simulink model "longitudinal_fuzzy_LiuChang"  (R2021b)
settings: Solver=VariableStepAuto  StartTime=0.0  StopTime=60  RelTol=1e-3
libraries: commrandsrc3 x3, fuzblock x3
settings Model: Creator=dell  LastModifiedBy=lenovo
settings SolverCC: ZeroCrossAlgorithm=Adaptive  AlgebraicLoopSolver=TrustRegion
settings DebuggingCC: IgnoredZcDiagnostic=none  SFMachineParentedDataDiag=warning  ArithmeticOperatorsInVariantConditions=warning
settings SFSimCC: CustomCodeUndefinedFunction=UseInterfaceOnly

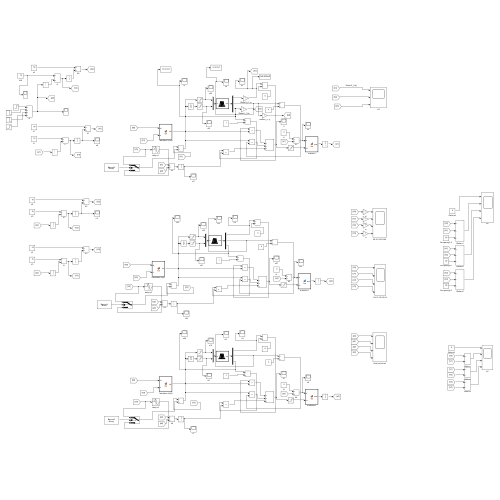
[thumbnail: Simulink's stored preview of the top-level diagram]
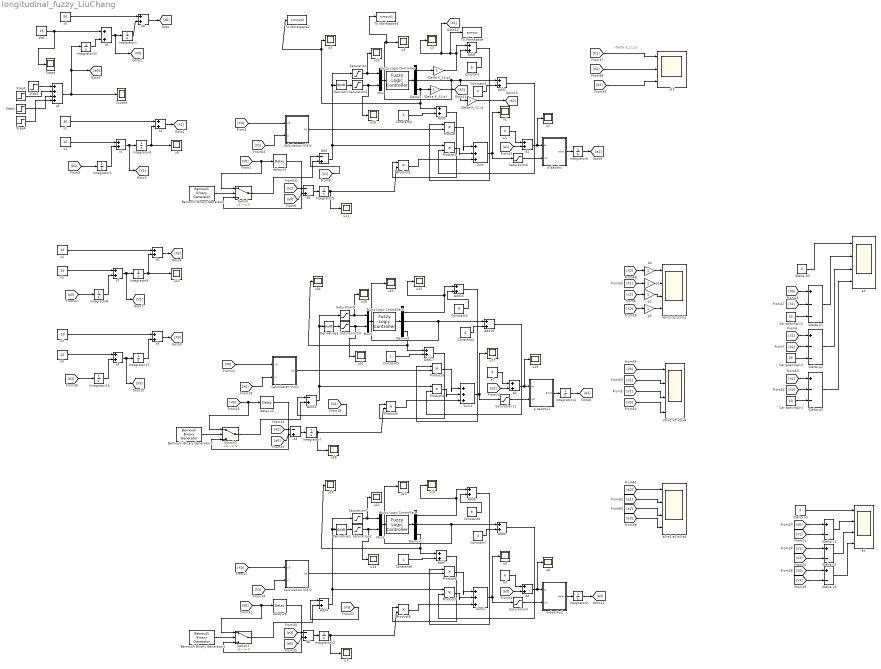
== system longitudinal_fuzzy_LiuChang ==
  note: \Delta K_{1,p}
  " Car spacing2-2" : Constant  Value=20
  " Car spacing2-3" : Constant  Value=20
  A1 : Sum
  A2 : Sum
  A3 : Sum  Inputs=-+
  A4 : Sum
  A5 : Sum  Inputs=-+
  A6 : Sum  Inputs=-+
  Add : Sum  Inputs=-+
  Add{1..3,5..7,15..17} (9 alike) : Sum
  Add14 : Sum  Inputs=-+
  Add4 : Sum  Inputs=-+
  Bernoulli Binary Generator : commrandsrc3/Bernoulli Binary Generator  ProbabilityOfZero=0.5  SeedSource=Auto  Seed=0  SampleTime=1  SamplesPerFrame=1  OutputDataType=double  SimulateUsing=Interpreted execution
  Bernoulli Binary Generator1 : commrandsrc3/Bernoulli Binary Generator  ProbabilityOfZero=0.5  SeedSource=Auto  Seed=0  SampleTime=1  SamplesPerFrame=1  OutputDataType=double  SimulateUsing=Interpreted execution
  Bernoulli Binary Generator3 : commrandsrc3/Bernoulli Binary Generator  ProbabilityOfZero=0.5  SeedSource=Auto  Seed=0  SampleTime=1  SamplesPerFrame=1  OutputDataType=double  SimulateUsing=Interpreted execution
  Calculation V(d)1 : MATLAB Function  TreatAsAtomicUnit=on
  Calculation V(d)2 : MATLAB Function  TreatAsAtomicUnit=on
  Calculation V(d)4 : MATLAB Function  TreatAsAtomicUnit=on
  Car spacing1-2 : Constant  Value=20
  Constant : Constant  Value=9
  Constant1 : Constant  Value=4
  Constant2 : Constant
  Constant3 : Constant  Value=9
  Constant4 : Constant  Value=4
  Constant5 : Constant
  Constant6 : Constant  Value=9
  Constant7 : Constant  Value=4
  Constant8 : Constant
  Demux : Demux  Outputs=3
  Demux1 : Demux  Outputs=3
  Demux3 : Demux  Outputs=3
  Derivative : Derivative
  Derivative1 : Derivative
  Derivative3 : Derivative
  Fuzzy Logic Controller : fuzblock/Fuzzy Logic  Controller  FIS='Fuzzy_longitudinal2.fis'  OutputSampleNumber=101  DataType=double  FuzzifiedInputs=off  RuleFiringStrengths=off  RuleOutputs=off  AggregatedOutputs=off  SimulateUsing=Interpreted execution  OutOfRangeInputValueMessage=warning  NoRuleFiredMessage=warning  EmptyOutputFuzzySetMessage=warning
  Fuzzy Logic Controller1 : fuzblock/Fuzzy Logic  Controller  FIS='Fuzzy_longitudinal2.fis'  OutputSampleNumber=101  DataType=double  FuzzifiedInputs=off  RuleFiringStrengths=off  RuleOutputs=off  AggregatedOutputs=off  SimulateUsing=Interpreted execution  OutOfRangeInputValueMessage=warning  NoRuleFiredMessage=warning  EmptyOutputFuzzySetMessage=warning
  Fuzzy Logic Controller3 : fuzblock/Fuzzy Logic  Controller  FIS='Fuzzy_longitudinal2.fis'  OutputSampleNumber=101  DataType=double  FuzzifiedInputs=off  RuleFiringStrengths=off  RuleOutputs=off  AggregatedOutputs=off  SimulateUsing=Interpreted execution  OutOfRangeInputValueMessage=warning  NoRuleFiredMessage=warning  EmptyOutputFuzzySetMessage=warning
  Integrator{1..12,16..17} (14 alike) : Integrator
  Mux : Mux  Inputs=2
  Mux1 : Mux  Inputs=2
  Mux3 : Mux  Inputs=2
  Product{,1..8} (9 alike) : Product
  Saturation{,1..2,7,9..10} (6 alike) : Saturate  UpperLimit=5  LowerLimit=-5  ZeroCross=off
  Saturation11 : Saturate  UpperLimit=5  LowerLimit=-5
  Saturation3 : Saturate  UpperLimit=5  LowerLimit=-5
  Saturation6 : Saturate  UpperLimit=5  LowerLimit=-5
  Scope : Scope
  Scope1 : Scope
  Step1 : Step  Time=30  After=-0.4  SampleTime=0
  Step2 : Step  Time=5  After=0.3  SampleTime=0
  Step3 : Step  Time=15  After=-0.3  SampleTime=0
  Step4 : Step  Time=40  After=0.4  SampleTime=0
  Sum : Sum  Inputs=|+++
  Sum1 : Sum  Inputs=|+++
  Sum2 : Sum  Inputs=|+++
  Switch : Switch  Criteria=u2 ~= 0
  Switch1 : Switch  Criteria=u2 ~= 0
  Switch3 : Switch  Criteria=u2 ~= 0
  To Workspace : ToWorkspace  VariableName=simout  SaveFormat=Timeseries  SampleTime=-1
  To Workspace1 : ToWorkspace  VariableName=simout1  SaveFormat=Timeseries  SampleTime=-1
  To Workspace2 : ToWorkspace  VariableName=simout2  SaveFormat=Timeseries  SampleTime=-1
  V0-V1-V2-V3-V4 : Scope  NumInputPorts=4
  V1 : Constant  Value=15
  V2 : Constant  Value=15
  V3 : Constant  Value=15
  VV0 : Constant  Value=15
  X{0..3} (4 alike) : Sum
  X0-X1-X2-X3-X4 : Scope  NumInputPorts=4
  "\\Delta K_{1,a}" : Gain
  "\\Delta K_{1,p}" : Gain
  "\\Delta K_{1,v}" : Gain
  \Delta p0 : Constant  Value=0
  \Delta p1 : Sum  Inputs=+--
  \Delta p2 : Sum  Inputs=+--
  \Delta p3 : Sum  Inputs=+--
  \Delta v0 : Constant  Value=0
  \Delta v1 : Sum  Inputs=+-
  \Delta v2 : Sum  Inputs=+-
  \Delta v3 : Sum  Inputs=+-
  a daoshu : MATLAB Function  TreatAsAtomicUnit=on
  a daoshu1 : MATLAB Function  TreatAsAtomicUnit=on
  a daoshu2 : MATLAB Function  TreatAsAtomicUnit=on
  a0-a1-a2-a3-a4 : Scope  NumInputPorts=4
  a1 : Constant  Value=0
  a2 : Constant  Value=0
  a3 : Constant  Value=0
  delay-v1 : TransportDelay  DelayTime=0.4
  delay-v2 : TransportDelay  DelayTime=0.4
  delay-v3 : TransportDelay  DelayTime=0.4
  eV : Scope  NumInputPorts=4
  eX : Scope  NumInputPorts=4
  p{0..3} (4 alike) : Gain
  u{1..14,23..34} (26 alike) : Scope
  u15 : Scope  NumInputPorts=3
  v{0..3} (4 alike) : Sum
  v6 : Sum  Inputs=++++
  x0 : Constant  Value=50
  x1 : Constant  Value=30
  x2 : Constant  Value=10
  x3 : Constant  Value=-10
  wires:
  v2/1 -> Integrator9/1, [V2]
  [X0] -> \Delta p1/1
  \Delta p2/1 -> eX/3
  A1/1 -> u2/1, a daoshu/1(ai)
  [X1] -> \Delta p2/1
  [V2] -> \Delta v2/2
  [a1] -> a0-a1-a2-a3-a4/2
  [X0] -> Calculation V(d)4/1(x0)
  \Delta v2/1 -> eV/3
  [a2] -> a0-a1-a2-a3-a4/3
  [V1] -> \Delta v1/2
  x3/1 -> X3/1
  [a3] -> a0-a1-a2-a3-a4/4
  [X2] -> \Delta p2/2
  A5/1 -> Integrator5/1
  [a0] -> A5/2
  [a0] -> a0-a1-a2-a3-a4/1
  a1/1 -> A1/1
  \Delta p0/1 -> eX/1
  \Delta p1/1 -> eX/2
  [V1] -> V0-V1-V2-V3-V4/2
  \Delta v1/1 -> eV/2
  Car spacing1-2/1 -> \Delta p1/3
  [V0] -> V0-V1-V2-V3-V4/1
  [X1] -> Calculation V(d)4/2(xi)
  x2/1 -> X2/1
  v1/1 -> Integrator4/1, [V1]
  [a3] -> Integrator16/1
  [V3] -> \Delta v3/2
  [V0] -> \Delta v1/1
  Sum/1 -> Saturation6/1, u1/1
  [V2] -> \Delta v3/1
  [X2] -> \Delta p3/1
  [V1] -> \Delta v2/1
  [a2] -> Integrator8/1
  " Car spacing2-2"/1 -> \Delta p3/3
  [V3] -> V0-V1-V2-V3-V4/4
  [a1] -> A5/1
  [V2] -> V0-V1-V2-V3-V4/3
  Integrator10/1 -> v0/2
  \Delta v0/1 -> eV/1
  \Delta v3/1 -> eV/4
  V3/1 -> v3/1
  [X3] -> \Delta p3/2
  [X1] -> \Delta p1/2
  " Car spacing2-3"/1 -> \Delta p2/3
  Integrator4/1 -> u9/1, X1/2
  X3/1 -> [X3]
  Integrator17/1 -> X3/2
  v3/1 -> Integrator17/1, [V3]
  Integrator16/1 -> v3/2
  X2/1 -> [X2]
  [a1] -> A1/2
  \Delta p3/1 -> eX/4
  Integrator8/1 -> v2/2
  V2/1 -> v2/1
  Integrator6/1 -> [a1]
  Integrator9/1 -> u10/1, X2/2
  v0/1 -> [V0], Integrator1/1
  [a1] -> Integrator3/1
  X1/1 -> [X1]
  Integrator3/1 -> v1/2
  x1/1 -> X1/1
  Integrator1/1 -> X0/2
  a daoshu/1(aout) -> Integrator6/1
  X0/1 -> [X0]
  x0/1 -> X0/1
  V1/1 -> v1/1
  VV0/1 -> Scope/1, v0/1
  Step2/1 -> v6/1
  Step3/1 -> v6/2
  v6/1 -> Scope1/1, [a0], Integrator10/1
  Step1/1 -> v6/3
  Step4/1 -> v6/4
  [V0] -> Switch/1, delay-v1/1
  [V1] -> Add/1
  Add/1 -> Product1/1, Saturation/1, Derivative/1
  Constant/1 -> Add1/2
  Fuzzy Logic Controller/1 -> Demux/1
  Mux/1 -> Fuzzy Logic Controller/1
  Derivative/1 -> Saturation1/1
  Saturation/1 -> u25/1, Mux/1
  Saturation1/1 -> u26/1, Mux/2
  Saturation6/1 -> a daoshu/2(uit)
  delay-v1/1 -> Switch/3
  Bernoulli Binary Generator/1 -> Switch/2
  Switch/1 -> Add/2
  Demux/1 -> "\\Delta K_{1,p}"/1
  Demux/2 -> To Workspace1/1, u4/1, "\\Delta K_{1,v}"/1, Add2/1
  Demux/3 -> To Workspace2/1, u5/1, Add3/1, "\\Delta K_{1,a}"/1
  Integrator5/1 -> u11/1, Product2/2
  Add1/1 -> Product/1
  Calculation V(d)4/1(Xd) -> Product/2
  Product/1 -> Sum/1
  Constant1/1 -> Add2/2
  Add2/1 -> Product1/2
  Product1/1 -> Sum/2
  Constant2/1 -> Add3/2
  Add3/1 -> Product2/1
  Product2/1 -> Sum/3
  Product4/1 -> Sum1/2
  Demux3/3 -> u34/1, Add17/1
  Saturation11/1 -> a daoshu1/2(uit)
  delay-v2/1 -> Switch3/3
  Add16/1 -> Product4/2
  Switch3/1 -> Add14/2
  Product5/1 -> Sum1/3
  Bernoulli Binary Generator3/1 -> Switch3/2
  [V0] -> Switch3/1, delay-v2/1
  a daoshu1/1(aout) -> Integrator11/1
  Saturation10/1 -> u31/1, Mux3/2
  [X2] -> Calculation V(d)1/2(xi)
  Derivative3/1 -> Saturation10/1
  Add14/1 -> Product4/1, Saturation9/1, Derivative3/1
  Saturation9/1 -> u30/1, Mux3/1
  Integrator7/1 -> u28/1, Product5/2
  Demux3/2 -> u33/1, Add16/1
  Fuzzy Logic Controller3/1 -> Demux3/1
  Mux3/1 -> Fuzzy Logic Controller3/1
  Demux3/1 -> Add15/1, u32/1
  [V2] -> Add14/1
  A2/1 -> u29/1, a daoshu1/1(ai)
  [a0] -> A3/2
  Constant5/1 -> Add17/2
  [a2] -> A3/1
  Sum1/1 -> Saturation11/1, u27/1
  Integrator11/1 -> [a2]
  Product3/1 -> Sum1/1
  A3/1 -> Integrator7/1
  Calculation V(d)1/1(Xd) -> Product3/2
  Add17/1 -> Product5/1
  Add15/1 -> Product3/1
  [X0] -> Calculation V(d)1/1(x0)
  Constant4/1 -> Add16/2
  Constant3/1 -> Add15/2
  a2/1 -> A2/1
  [a2] -> A2/2
  Add4/1 -> Product7/1, Saturation7/1, Derivative1/1
  [X3] -> Calculation V(d)2/2(xi)
  a daoshu2/1(aout) -> Integrator2/1
  Product8/1 -> Sum2/3
  Switch1/1 -> Add4/2
  Bernoulli Binary Generator1/1 -> Switch1/2
  Saturation3/1 -> a daoshu2/2(uit)
  Derivative1/1 -> Saturation2/1
  A6/1 -> Integrator12/1
  Calculation V(d)2/1(Xd) -> Product6/2
  [X0] -> Calculation V(d)2/1(x0)
  Fuzzy Logic Controller1/1 -> Demux1/1
  Mux1/1 -> Fuzzy Logic Controller1/1
  Integrator2/1 -> [a3]
  Integrator12/1 -> u7/1, Product8/2
  Demux1/1 -> Add5/1, u14/1
  a3/1 -> A4/1
  [a3] -> A4/2
  Constant7/1 -> Add6/2
  Demux1/3 -> u24/1, Add7/1
  Saturation7/1 -> u12/1, Mux1/1
  Constant6/1 -> Add5/2
  [a3] -> A6/1
  Add7/1 -> Product8/1
  [a0] -> A6/2
  Product6/1 -> Sum2/1
  Add5/1 -> Product6/1
  Product7/1 -> Sum2/2
  [V3] -> Add4/1
  Constant8/1 -> Add7/2
  Sum2/1 -> Saturation3/1, u6/1
  [V0] -> Switch1/1, delay-v3/1
  Add6/1 -> Product7/2
  delay-v3/1 -> Switch1/3
  A4/1 -> u8/1, a daoshu2/1(ai)
  Demux1/2 -> u23/1, Add6/1
  Saturation2/1 -> u13/1, Mux1/2
  [K1] -> u15/1
  [K3] -> u15/3
  [K2] -> u15/2
  "\\Delta K_{1,p}"/1 -> Add1/1, To Workspace/1, [K1], u3/1
  "\\Delta K_{1,v}"/1 -> [K2]
  "\\Delta K_{1,a}"/1 -> [K3]
  [X0] -> p0/1
  p0/1 -> X0-X1-X2-X3-X4/1
  [X1] -> p1/1
  p1/1 -> X0-X1-X2-X3-X4/2
  [X2] -> p2/1
  p2/1 -> X0-X1-X2-X3-X4/3
  [X3] -> p3/1
  p3/1 -> X0-X1-X2-X3-X4/4

== matlab function longitudinal_fuzzy_LiuChang/Calculation V(d)1 ==
  data: x0 input; Xd output; xi input
  function Xd  = fcn(x0,xi)
Xd=x0-xi-40;
  end

== matlab function longitudinal_fuzzy_LiuChang/Calculation V(d)4 ==
  data: x0 input; Xd output; xi input
  function Xd  = fcn(x0,xi)
Xd=x0-xi-20;
  end

== matlab function longitudinal_fuzzy_LiuChang/a daoshu1 ==
  data: ai input; aout output; uit input
function aout  = fcn(ai,uit)
b=0.1;
aout=1/b*uit-1/b*ai;

end

== matlab function longitudinal_fuzzy_LiuChang/Calculation V(d)2 ==
  data: x0 input; Xd output; xi input
  function Xd  = fcn(x0,xi)
Xd=x0-xi-60;
  end

== matlab function longitudinal_fuzzy_LiuChang/a daoshu2 ==
  data: ai input; aout output; uit input
function aout  = fcn(ai,uit)
b=0.1;
aout=1/b*uit-1/b*ai;

end

== matlab function longitudinal_fuzzy_LiuChang/a daoshu ==
  data: ai input; aout output; uit input
function aout  = fcn(ai,uit)
b=0.1;
aout=1/b*uit-1/b*ai;

end
